simulink model "GEB"  (R2020a)
settings: Solver=FixedStepAuto  StartTime=20478600  StopTime=20479500+60*15  FixedStep=60*15  RelTol=1e-3
undefined symbols (not defined in the file or in its folder): Discrete, Time
libraries: ctrlSharedLib x1
settings Model: Creator=Aaron  LastModifiedBy=yl3328

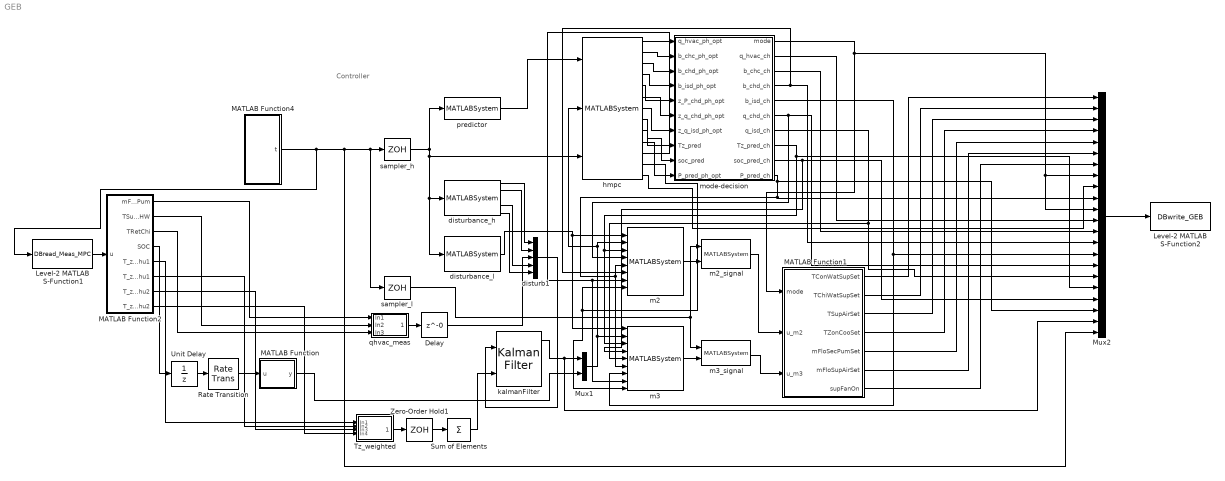
== system GEB ==
  note: Controller
  Delay : Delay  DelayLength=0  SampleTime=3600
  Level-2 MATLAB S-Function1 : M-S-Function  FunctionName=DBread_Meas_MPC
  Level-2 MATLAB S-Function2 : M-S-Function  FunctionName=DBwrite_GEB
  MATLAB Function : MATLAB Function  TreatAsAtomicUnit=on
  MATLAB Function1 : MATLAB Function  TreatAsAtomicUnit=on
  MATLAB Function2 : MATLAB Function  TreatAsAtomicUnit=on
  MATLAB Function4 : MATLAB Function  TreatAsAtomicUnit=on
  Mux1 : Mux  Inputs=2
  Mux2 : Mux  Inputs=22
  Rate Transition : RateTransition  InitialCondition=0.7  OutPortSampleTime=3600
  Sum of Elements : Sum  Inputs=+
  Tz_weighted : Subsystem
  Unit Delay : UnitDelay  InitialCondition=0.7  SampleTime=-1  HasFrameUpgradeWarning=on
  Zero-Order Hold1 : ZeroOrderHold  SampleTime=3600
  disturb1 : Concatenate  NumInputs=5
  disturbance_h : MATLABSystem  System=get_predictors_block_kalman  PH=1  CH=1  dt=3600  np=5  SimulateUsing=Interpreted execution
      mask Type: get_predictors_block_kalman
      mask Display:
      | disp('get_predictors_block_kalman');
      | port_label('input',1,'time');
      | port_label('output',1,'out1');
      | port_label('output',2,'out2');
      | port_label('output',3,'out3');
      | port_label('output',4,'out4');
      | port_label('output',5,'out5');
  disturbance_l : MATLABSystem  System=get_predictors_block_15min  PH=4  CH=1  dt=900  np=5  SimulateUsing=Interpreted execution
      mask Type: get_predictors_block_15min
      mask Display:
      | disp('get_predictors_block_15min');
      | port_label('input',1,'time');
      | port_label('output',1,'predictors');
  hmpc : MATLABSystem  System=hmpc_casadi_block_minlp  PH=24  CH=1  dt=3600  E_is_max=333.550 * 2846.35  q_chd_nom=26.4  q_chc_nom=18.970  cop_nom=4.55  number_zone=1  occ_start=7  occ_end=20  nu=13  soc_min=0.3  soc_max=1.0  w=[ 1, 1000, 0]  q_isd_min=0.01 * 104.220  q_isd_max=104.220  price_tou=[0.0298, 0.0298, 0.0298, 0.0298, 0.0298, 0.0298, 0.0298, 0.0409, 0.0409, 0.0409, 0.113, 0.113, 0.113, 0.113, 0.113, 0.113, 0.0409, 0.0409, 0.0409, 0.0298, 0.0298, 0.0298, 0.0298, 0.0298]  m_oa_ahu1=0.295  m_oa_ahu2=0.142  q_oa_max=10  cpa=1.01  SimulateUsing=Interpreted execution
      mask Type: hmpc_casadi_block_minlp
      mask Display:
      | disp('hmpc_casadi_block_minlp');
      | port_label('input',1,'predictor');
      | port_label('input',2,'states');
      | port_label('input',3,'time');
      | port_label('output',1,'q_hvac_ph_opt');
      | port_label('output',2,'b_chc_ph_opt');
      | port_label('output',3,'b_chd_ph_opt');
      | port_label('output',4,'b_isd_ph_opt');
      | port_label('output',5,'z_P_chd_ph_opt');
      | port_label('output',6,'z_q_chd_ph_opt');
      | port_label('output',7,'z_q_isd_ph_opt');
      | port_label('output',8,'Tz_pred');
      | port_label('output',9,'soc_pred');
      | port_label('output',10,'P_pred_ph_opt');
      | port_label('output',11,'z_q_oa_ph_opt');
      | port_label('output',12,'m_oa_ph_opt');
      | port_label('output',13,'optimalFlag');
  kalmanFilter : ctrlSharedLib/Kalman Filter  TimeDomain=Discrete-Time  UseCurrentEstimator=on  ModelSource=Individual A, B, C, D matrices  ModelSourceVariable=ss(0.95,1,1,0,1)  A=[-0.0694, 0, 0.9397; 0, 0.8592, 0.0296; 0.0347, 0.0034, 0.9619]  B=[0.1296, 0.5177,0.5177, 0 ,0; 0.1113, 0,0,0.1669,0;0,0,0,0,0.0191]  C=[1, 0, 0]  D=0  NumberOfStates=1  NumberOfInputs=1  NumberOfOutputs=1  InitialEstimateSource=Dialog  X0=[32.0592, 20.3112, 31.1369]  P0=10  UseK=off  UseGH=off  NumberOfProcessNoiseInputs=1  G=[1,0;0,1;1,0;0,1]  TimeInvariantG=on  H=0  TimeInvariantH=on  Q=diag([1, 1, 1])  TimeInvariantQ=on  R=0.5  TimeInvariantR=on  N=0  TimeInvariantN=on  AddInputPort=on  AddEnablePort=off  OutputEstimatedY=on  OutputP=on  Ts=-1
  m2 : MATLABSystem  System=m2_chiller_discharging_opc  dt=900  mpchwp_max=1.30  q_chd_max=26.4  PLR_min=0.3  PLR_max=1  Cpw=3.915  Cpa=1.081  nu=9  M=4  u_lb=[ 29.44, 5, 12, 8, 0, 0.9477, 0.1 * 26.400, 0, 0 ]  u_ub=[ 29.44, 10, 40, 12, 0.9748, 1.89, 1 *26.400, 0.1, 0.01 ]  w=[ 1.0, 100.0 ]  q_small=10  SimulateUsing=Interpreted execution
      mask Type: m2_chiller_discharging_opc
      mask Display:
      | disp('m2_chiller_discharging_opc');
      | port_label('input',1,'predictor');
      | port_label('input',2,'states');
      | port_label('input',3,'Tz_h');
      | port_label('input',4,'q_chd_h');
      | port_label('input',5,'P_h');
      | port_label('input',6,'on');
      | port_label('input',7,'q_oa_h');
      | port_label('input',8,'m_oa_h');
      | port_label('output',1,'u_opt_resh');
  m2_signal : MATLABSystem  System=transfer2signal  dt_h=3600  dt_l=900  nu=6  SimulateUsing=Code generation
      mask Type: transfer2signal
      mask Display:
      | disp('transfer2signal');
      | port_label('input',1,'time');
      | port_label('input',2,'u');
      | port_label('output',1,'ui');
  m3 : MATLABSystem  System=m3_tank_discharging_opc  dt=900  mpchwp_max=2.25  q_isd_max=100.000  E_is_max=333.550 * 2846.35  PLR_min=0.01  PLR_max=1.0  SOC_min=0.3  SOC_max=1.0  Cpw=3.915  Cpa=1.081  nu=9  M=4  u_lb=[ 5, 12, 6, 0.5849, 0.9477, 0.01 * 100.00, 0, 0, 0 ]  u_ub=[ 10, 40, 12, 1.7547, 1.89, 1.1 * 100.00, 0.1, 0.01, 0.01 ]  w=[ 10.0, 100.0, 1e6 ]  q_small=10  SimulateUsing=Interpreted execution
      mask Type: m3_tank_discharging_opc
      mask Display:
      | disp('m3_tank_discharging_opc');
      | port_label('input',1,'predictor');
      | port_label('input',2,'states');
      | port_label('input',3,'Tz_h');
      | port_label('input',4,'SOC_h');
      | port_label('input',5,'q_isd_h');
      | port_label('input',6,'P_h');
      | port_label('input',7,'on');
      | port_label('input',8,'q_oa_h');
      | port_label('input',9,'m_oa_h');
      | port_label('output',1,'u_opt_resh');
  m3_signal : MATLABSystem  System=transfer2signal  dt_h=3600  dt_l=900  nu=5  SimulateUsing=Code generation
      mask Type: transfer2signal
      mask Display:
      | disp('transfer2signal');
      | port_label('input',1,'time');
      | port_label('input',2,'u');
      | port_label('output',1,'ui');
  mode-decision : MATLAB Function  TreatAsAtomicUnit=on
  predictor : MATLABSystem  System=get_predictors_block  PH=24  CH=1  dt=3600  np=5  SimulateUsing=Interpreted execution
      mask Type: get_predictors_block
      mask Display:
      | disp('get_predictors_block');
      | port_label('input',1,'time');
      | port_label('output',1,'predictors');
  qhvac_meas : Subsystem
  sampler_h : ZeroOrderHold  SampleTime=3600
  sampler_l : ZeroOrderHold  SampleTime=900
  wires:
  m2_signal/1 -> MATLAB Function1/2(u_m2)
  MATLAB Function2/3(TRetChi) -> qhvac_meas/3(In3)
  MATLAB Function2/2(TSupCHW) -> qhvac_meas/2(In2)
  m3_signal/1 -> MATLAB Function1/3(u_m3)
  mode-decision/8(Tz_pred_ch) -> Mux2/18, m3/3, m2/3
  Sum of Elements/1 -> kalmanFilter/2
  sampler_l/1 -> m3_signal/1, m2_signal/1
  hmpc/4 -> mode-decision/4(b_isd_ph_opt)
  disturbance_l/1 -> m3/1, m2/1
  mode-decision/9(soc_pred_ch) -> Mux2/19, m3/4
  Delay/1 -> disturb1/3
  hmpc/1 -> mode-decision/1(q_hvac_ph_opt)
  disturbance_h/1 -> disturb1/1
  sampler_h/1 -> disturbance_l/1, disturbance_h/1, hmpc/3, predictor/1
  mode-decision/7(q_isd_ch) -> Mux2/17, m3/5
  hmpc/6 -> mode-decision/6(z_q_chd_ph_opt)
  m2/1 -> m2_signal/2
  mode-decision/6(q_chd_ch) -> Mux2/16, m2/4
  mode-decision/5(b_isd_ch) -> Mux2/15, m3/7
  kalmanFilter/1 -> Mux2/21, Mux1/1
  hmpc/3 -> mode-decision/3(b_chd_ph_opt)
  Tz_weighted/1(Out1) -> Zero-Order Hold1/1
  disturbance_h/5 -> disturb1/5
  disturbance_h/2 -> disturb1/2
  predictor/1 -> hmpc/1
  MATLAB Function2/1(mFloSecPum) -> qhvac_meas/1(In1)
  qhvac_meas/1(Out1) -> Delay/1
  hmpc/10 -> mode-decision/10(P_pred_ph_opt)
  disturb1/1 -> kalmanFilter/1
  m3/1 -> m3_signal/2
  mode-decision/4(b_chd_ch) -> Mux2/14, m2/6
  hmpc/5 -> mode-decision/5(z_P_chd_ph_opt)
  hmpc/8 -> mode-decision/8(Tz_pred)
  Zero-Order Hold1/1 -> Sum of Elements/1
  hmpc/9 -> mode-decision/9(soc_pred)
  Mux1/1 -> m2/2, hmpc/2, m3/2
  disturbance_h/4 -> disturb1/4
  hmpc/2 -> mode-decision/2(b_chc_ph_opt)
  hmpc/7 -> mode-decision/7(z_q_isd_ph_opt)
  mode-decision/1(mode) -> Mux2/11, Mux2/8, MATLAB Function1/1(mode)
  Mux2/1 -> Level-2 MATLAB S-Function2/1
  MATLAB Function1/1(TConWatSupSet) -> Mux2/1
  MATLAB Function1/2(TChiWatSupSet) -> Mux2/2
  MATLAB Function1/3(TSupAirSet) -> Mux2/3
  MATLAB Function1/4(TZonCooSet) -> Mux2/4
  MATLAB Function1/5(mFloSecPumSet) -> Mux2/5
  MATLAB Function1/6(mFloSupAirSet) -> Mux2/6
  MATLAB Function1/7(supFanOn) -> Mux2/7
  Level-2 MATLAB S-Function1/1 -> MATLAB Function2/1(u)
  MATLAB Function4/1(t) -> Level-2 MATLAB S-Function1/1, Mux2/22, sampler_l/1, sampler_h/1
  Unit Delay/1 -> Rate Transition/1
  MATLAB Function2/4(SOC) -> Unit Delay/1
  Rate Transition/1 -> MATLAB Function/1(u)
  MATLAB Function/1(y) -> Mux1/2
  MATLAB Function2/5(T_z1_ahu1) -> Tz_weighted/1(In1)
  MATLAB Function2/6(T_z2_ahu1) -> Tz_weighted/2(In2)
  MATLAB Function2/7(T_z1_ahu2) -> Tz_weighted/3(In3)
  MATLAB Function2/8(T_z2_ahu2) -> Tz_weighted/4(In4)
  mode-decision/10(P_pred_ch) -> Mux2/20, Mux2/10, m3/6, m2/5
  mode-decision/2(q_hvac_ch) -> Mux2/12
  mode-decision/3(b_chc_ch) -> Mux2/13
  hmpc/13 -> Mux2/9
  hmpc/11 -> m2/7, m3/8
  hmpc/12 -> m3/9, m2/8

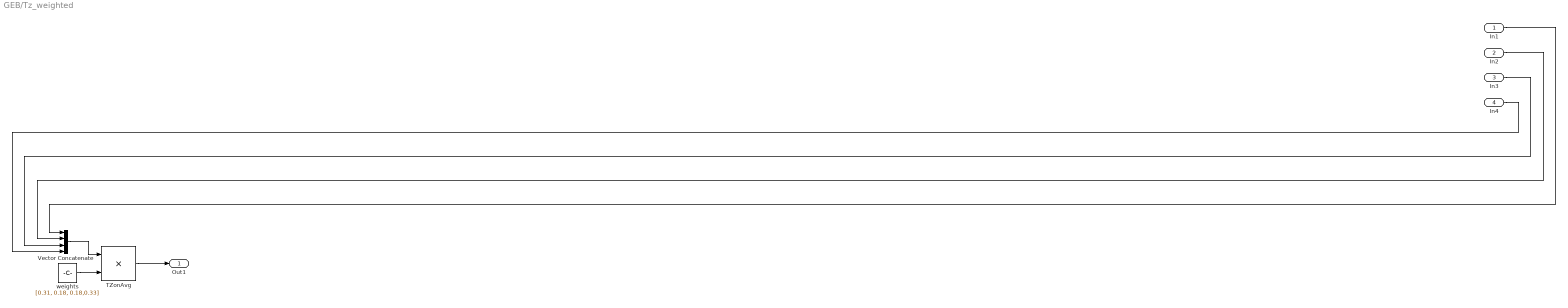
== system GEB/Tz_weighted ==
  In1 : Inport
  In2 : Inport  Port=2
  In3 : Inport  Port=3
  In4 : Inport  Port=4
  TZonAvg : Product
  Vector Concatenate : Concatenate  NumInputs=4
  weights : Constant  Value=[0.31, 0.18, 0.18,0.33]
  Out1 : Outport
  wires:
  In1/1 -> Vector Concatenate/1
  Vector Concatenate/1 -> TZonAvg/1
  In3/1 -> Vector Concatenate/3
  In4/1 -> Vector Concatenate/4
  TZonAvg/1 -> Out1/1
  weights/1 -> TZonAvg/2
  In2/1 -> Vector Concatenate/2

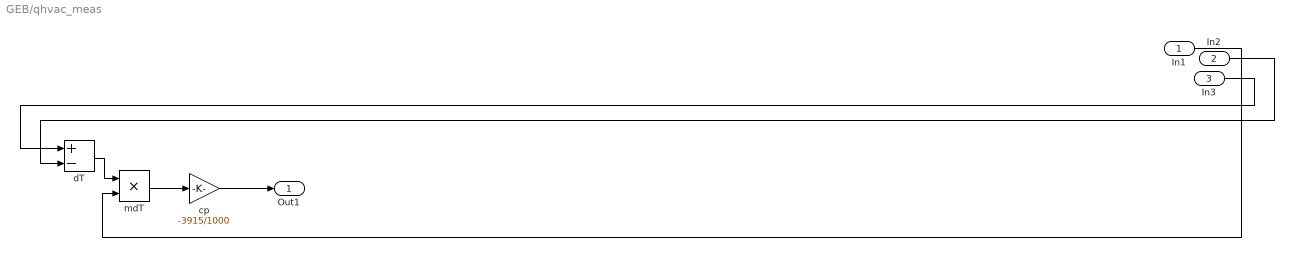
== system GEB/qhvac_meas ==
  In1 : Inport
  In2 : Inport  Port=2
  In3 : Inport  Port=3
  cp : Gain  Gain=-3915/1000
  dT : Sum  Inputs=+-
  mdT : Product
  Out1 : Outport
  wires:
  In3/1 -> dT/1
  dT/1 -> mdT/1
  mdT/1 -> cp/1
  In2/1 -> dT/2
  In1/1 -> mdT/2
  cp/1 -> Out1/1

== matlab function GEB/MATLAB Function1 ==
  data: TConWatSupSet output; TChiWatSupSet output; TSupAirSet output; TZonCooSet output; mFloSecPumSet output; mFloSupAirSet output; mode input; supFanOn output; u_m2 input; u_m3 input
function [TConWatSupSet, TChiWatSupSet, TSupAirSet, TZonCooSet, mFloSecPumSet, mFloSupAirSet,supFanOn] = SignalToTestbed(mode, u_m2, u_m3)
% INPUTS:
%   mode: operation mode: 1: off, 2: discharge tank and chiller, 3: discharge tank, 4: discharge chiller, 5: charge tank
%   u_m2: nu2-by-1: control signal for m2: [Tcw_opt;Tchw_opt;Tsa_opt;Tz_pred; mschwp_opt; msa_opt];
%   u_m3: nu3-by-1: control signal for m3: [Tchw_opt;Tsa_opt;Tz_pred; mschwp_opt; msa_opt]
% OUTPUTS:
%   TConWatSupSet, TChiWatSupSet, TSupAirSet, TZonCooSet, mFloSecPumSet,
%   mFlowSupAirSet, supFanOn

% supply fan on/off
supFanOn = 1;
if mode==1 || mode==5
    supFanOn = 0;
end

% condenser water 
TConWatSupSet = u_m2(1) + 273.15;

% chilled water 
TChiWatSupSet = u_m2(2) + 273.15;
if mode==3
    TChiWatSupSet = u_m3(1) + 273.15;
end

% supply air temperature
TSupAirSet = u_m2(3) + 273.15;
if mode==3
    TSupAirSet = u_m3(2) + 273.15;
end

% zone temperature set
TZonCooSet = u_m2(4) + 273.15;
if mode==3
    TZonCooSet = u_m3(3) + 273.15;
end
% secondary pump flow
mFloSecPumSet = u_m2(5);
if mode==3
    mFloSecPumSet = u_m3(4);
end

% supply air flow set
mFloSupAirSet = u_m2(6);
if mode==3
    mFloSupAirSet = u_m3(5);
end
end

== matlab function GEB/MATLAB Function2 ==
  data: mFloSecPum output; u input; TSupCHW output; TRetChi output; SOC output; T_z1_ahu1 output; T_z2_ahu1 output; T_z1_ahu2 output; T_z2_ahu2 output
function [mFloSecPum, TSupCHW, TRetChi, SOC, T_z1_ahu1, T_z2_ahu1, T_z1_ahu2, T_z2_ahu2] = fcn(u)

coder.extrinsic('xlsread');
TES=0;
[TES] = xlsread('settings.csv', 1,'G2');

mFloSecPum = zeros(1);
TSupCHW = zeros(1);
TRetChi = zeros(1);
SOC = zeros(1);
T_z1_ahu1 = zeros(1);
T_z2_ahu1 = zeros(1);
T_z1_ahu2 = zeros(1);
T_z2_ahu2 = zeros(1);

mFloSecPum=u(1);
TSupCHW=u(2);
TRetChi=u(3);
SOC=u(4);
% for TES cases, add a constraint that TES inventory must higher than 50%
if SOC<0.5 && TES==0
    SOC=0.5;
end

T_z1_ahu1=u(5);
T_z2_ahu1=u(6);
T_z1_ahu2=u(7);
T_z2_ahu2=u(8);

== matlab function GEB/mode-decision ==
  data: q_hvac_ph_opt input; mode output; b_chc_ph_opt input; b_chd_ph_opt input; b_isd_ph_opt input; z_P_chd_ph_opt input; z_q_chd_ph_opt input; z_q_isd_ph_opt input; Tz_pred input; soc_pred input; P_pred_ph_opt input; q_hvac_ch output; b_chc_ch output; b_chd_ch output; b_isd_ch output; q_chd_ch output; q_isd_ch output; Tz_pred_ch output; soc_pred_ch output; P_pred_ch output
function [mode, q_hvac_ch, b_chc_ch, b_chd_ch, b_isd_ch, q_chd_ch, q_isd_ch, Tz_pred_ch, soc_pred_ch, P_pred_ch] = fcn(q_hvac_ph_opt, b_chc_ph_opt,...
                  b_chd_ph_opt, b_isd_ph_opt, z_P_chd_ph_opt, ...
                  z_q_chd_ph_opt, z_q_isd_ph_opt, Tz_pred, ...
                  soc_pred, P_pred_ph_opt)
% calculate output
q_hvac_ch = q_hvac_ph_opt(1);
b_chc_ch = b_chc_ph_opt(1);
b_chd_ch = b_chd_ph_opt(1);
b_isd_ch = b_isd_ph_opt(1);
q_chd_ch = z_q_chd_ph_opt(1);
q_isd_ch = z_q_isd_ph_opt(1);
Tz_pred_ch = Tz_pred(1);
soc_pred_ch = soc_pred(1);
P_pred_ch = P_pred_ph_opt(1);

% get cooling mode
% "1: off, 2: discharge tank and chiller, 3: discharge tank, 4: discharge chiller, 5: charge tank"
mode = 1;
if b_chc_ch > 0.5
    mode = 5;
elseif b_chd_ch > 0.5 && b_isd_ch < 0.5
    mode = 4;
elseif b_chd_ch < 0.5 && b_isd_ch > 0.5
    mode = 3;
else
    mode = 1;
end

end

== matlab function GEB/MATLAB Function4 ==
  data: t output
function t  = fcn
coder.extrinsic('xlsread');
T=0;
[T] = xlsread('Time.xlsx', 1,'B1');
t=0;
t=T+60*15;

== matlab function GEB/MATLAB Function ==
  data: u input; y output
function y = fcn(u)

y = u;
